simulink model "Inputs"  (R2018b)
settings: configuration reference "FixedStepConfiguration" (kept outside this file)
libraries: arduinolib x3
settings Model: DataDictionary=DataDictionary.sldd  Creator=chris  LastModifiedBy=chris

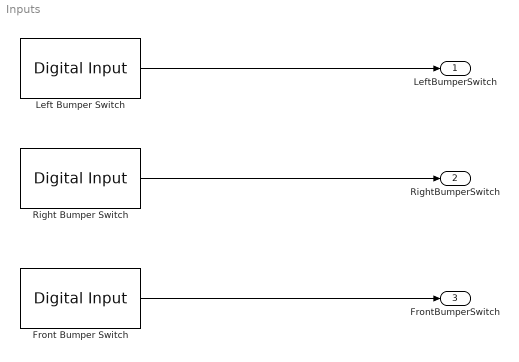
== system Inputs ==
  Front Bumper Switch : arduinolib/Digital Input  pinNumber=10  sampleTime=0.1  blockPlatform=arduino
      settings: SourceProductName=Simulink Support Package for Arduino Hardware
  Left Bumper Switch : arduinolib/Digital Input  pinNumber=8  sampleTime=0.1  blockPlatform=arduino
      settings: SourceProductName=Simulink Support Package for Arduino Hardware
  Right Bumper Switch : arduinolib/Digital Input  pinNumber=9  sampleTime=0.1  blockPlatform=arduino
      settings: SourceProductName=Simulink Support Package for Arduino Hardware
  LeftBumperSwitch : Outport
  RightBumperSwitch : Outport  Port=2
  FrontBumperSwitch : Outport  Port=3
  wires:
  Right Bumper Switch/1 -> RightBumperSwitch/1
  Left Bumper Switch/1 -> LeftBumperSwitch/1
  Front Bumper Switch/1 -> FrontBumperSwitch/1
